simulink model "cvoo_g19_sae"  (R2020a)
settings: Solver=VariableStepAuto  StartTime=0.0  StopTime=10.0  RelTol=1e-3
values from neighbouring files (symbols this model uses):
  a_h = [ ... (first row only)    [Ponto2.m]
  b_h_sf = b_h(:,[1,3])    [Ponto2.m]
  c_h = eye(size(a_h))    [Ponto2.m]
  d_h_sf = d_h(:,[1,3])    [Ponto2.m]
  de_step = 1*pi/180    (= 0.0174532925199)    [Ponto2.m]
  dsp_step = 10*pi/180    (= 0.174532925199)    [Ponto2.m]
  k_u_dsp = 0.65    [Ponto2.m]
  k_w_dsp = 4.1    [Ponto2.m]
  t_de_ini = 1    [Ponto2.m]
  t_de_step = 2    [Ponto2.m]
  t_dsp_ini = 50    [Ponto2.m]
  t_dsp_step = 10    [Ponto2.m]
  x0_h = [0 0 0 0 0]    [Ponto2.m]
undefined symbols (not defined in the file or in its folder): cond_ini
settings Model: Creator=josem  LastModifiedBy=josem

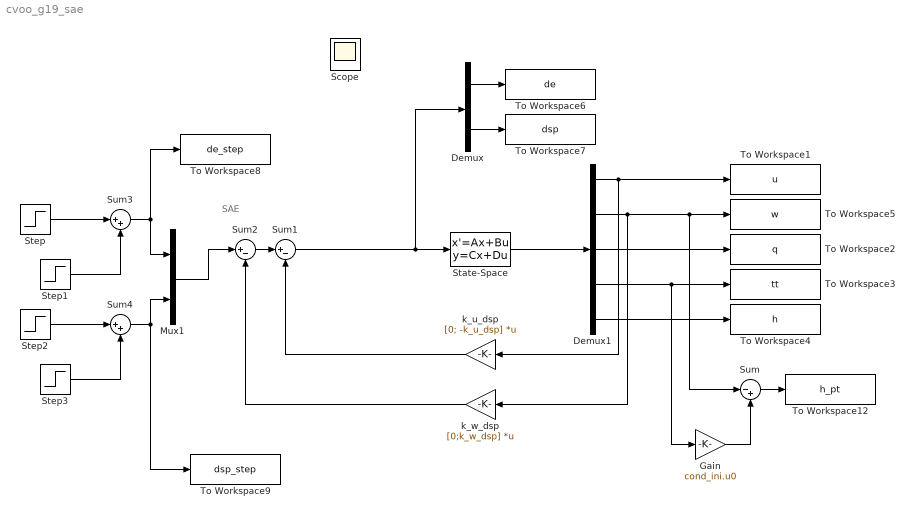
== system cvoo_g19_sae ==
  note: SAE
  Demux : Demux  Outputs=2
  Demux1 : Demux  Outputs=5
  Gain : Gain  Gain=cond_ini.u0
  Mux1 : Mux  Inputs=2
  State-Space : StateSpace  A=a_h  B=b_h_sf  C=c_h  D=d_h_sf  InitialCondition=x0_h
  Step : Step  Time=t_de_ini  After=de_step  SampleTime=0
  Step1 : Step  Time=t_de_ini+t_de_step  After=-de_step  SampleTime=0
  Step2 : Step  Time=t_dsp_ini  After=dsp_step  SampleTime=0
  Step3 : Step  Time=t_dsp_ini+t_dsp_step  After=-dsp_step  SampleTime=0
  Sum : Sum  Inputs=|-+
  Sum1 : Sum  Inputs=|+-
  Sum2 : Sum  Inputs=|+-
  Sum3 : Sum  Inputs=|++
  Sum4 : Sum  Inputs=|++
  To Workspace1 : ToWorkspace  VariableName=u  SampleTime=-1
  To Workspace12 : ToWorkspace  VariableName=h_pt  SampleTime=-1
  To Workspace2 : ToWorkspace  VariableName=q  SampleTime=-1
  To Workspace3 : ToWorkspace  VariableName=tt  SampleTime=-1
  To Workspace4 : ToWorkspace  VariableName=h  SampleTime=-1
  To Workspace5 : ToWorkspace  VariableName=w  SampleTime=-1
  To Workspace6 : ToWorkspace  VariableName=de  SampleTime=-1
  To Workspace7 : ToWorkspace  VariableName=dsp  SampleTime=-1
  To Workspace8 : ToWorkspace  VariableName=de_step  SampleTime=-1
  To Workspace9 : ToWorkspace  VariableName=dsp_step  SampleTime=-1
  k_u_dsp : Gain  Gain=[0; -k_u_dsp]  Multiplication=Matrix(K*u)
  k_w_dsp : Gain  Gain=[0;k_w_dsp]  Multiplication=Matrix(K*u)
  Scope : Scope
  wires:
  State-Space/1 -> Demux1/1
  Demux1/1 -> k_u_dsp/1, To Workspace1/1
  Demux1/3 -> To Workspace2/1
  Demux1/4 -> To Workspace3/1, Gain/1
  Demux1/5 -> To Workspace4/1
  k_u_dsp/1 -> Sum1/2
  Sum2/1 -> Sum1/1
  k_w_dsp/1 -> Sum2/2
  Demux/1 -> To Workspace6/1
  Demux/2 -> To Workspace7/1
  Step/1 -> Sum3/1
  Step1/1 -> Sum3/2
  Mux1/1 -> Sum2/1
  Sum3/1 -> To Workspace8/1, Mux1/1
  Step2/1 -> Sum4/1
  Step3/1 -> Sum4/2
  Sum4/1 -> To Workspace9/1, Mux1/2
  Sum1/1 -> Demux/1, State-Space/1
  Demux1/2 -> k_w_dsp/1, Sum/1, To Workspace5/1
  Gain/1 -> Sum/2
  Sum/1 -> To Workspace12/1
